simulink model "phan1_bai2a_kieu1_2016a"  (R2016a)
settings: Solver=VariableStepAuto  SolverMode=SingleTasking  StartTime=0.0  StopTime=30  RelTol=1e-3
libraries: simulink x1
settings Model: Creator=inhuo  LastModifiedBy=inhuo
settings DataIOCC: ReturnWorkspaceOutputs=on
settings DebuggingCC: SFUnexpectedBacktrackingDiag=error  SFNoUnconditionalDefaultTransitionDiag=error
settings SFSimCC: SimUseLocalCustomCode=on
settings RTWCC: RTWUseLocalCustomCode=on
settings GRTTargetCC: TargetLangStandard=C99 (ISO)  GeneratePreprocessorConditionals=Use local settings
settings ConfigComp: CovMetricSettings=dwe  CovHtmlReporting=off  CovSaveCumulativeToWorkspaceVar=off  CovSaveSingleToWorkspaceVar=off  CovExternalEMLEnable=on

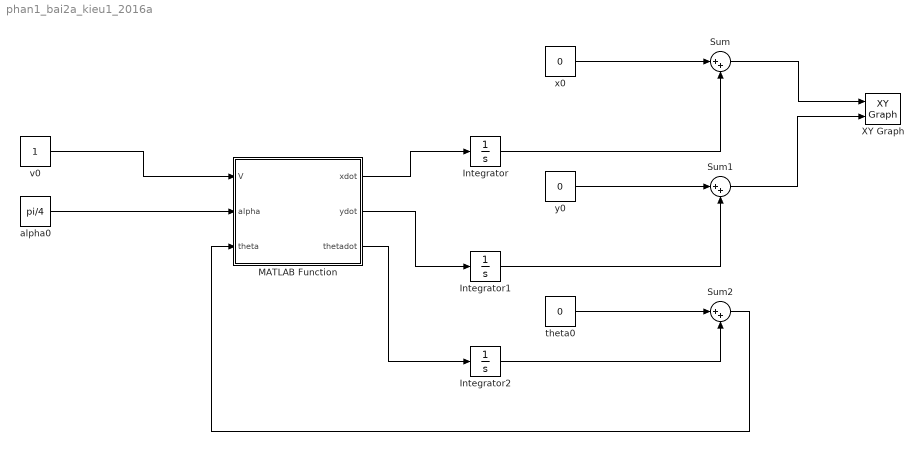
== system phan1_bai2a_kieu1_2016a ==
  Integrator : Integrator
  Integrator1 : Integrator
  Integrator2 : Integrator
  MATLAB Function : MATLAB Function  TreatAsAtomicUnit=on
  Sum : Sum  Inputs=|++
  Sum1 : Sum  Inputs=|++
  Sum2 : Sum  Inputs=|++
  XY Graph : simulink/Sinks/XY Graph  xmin=-5  xmax=10  ymin=-5  ymax=10  st=-1
  alpha0 : Constant  Value=pi/4
  theta0 : Constant  Value=0
  v0 : Constant
  x0 : Constant  Value=0
  y0 : Constant  Value=0
  wires:
  Sum2/1 -> MATLAB Function/3(theta)
  v0/1 -> MATLAB Function/1(V)
  MATLAB Function/2(ydot) -> Integrator1/1
  Sum/1 -> XY Graph/1
  Integrator1/1 -> Sum1/2
  MATLAB Function/3(thetadot) -> Integrator2/1
  x0/1 -> Sum/1
  Sum1/1 -> XY Graph/2
  theta0/1 -> Sum2/1
  Integrator2/1 -> Sum2/2
  y0/1 -> Sum1/1
  alpha0/1 -> MATLAB Function/2(alpha)
  MATLAB Function/1(xdot) -> Integrator/1
  Integrator/1 -> Sum/2

== matlab function phan1_bai2a_kieu1_2016a/MATLAB Function ==
  data: V input; xdot output; alpha input; theta input; ydot output; thetadot output
function [xdot , ydot , thetadot]= fcn(V,alpha,theta)

    d = sqrt (2.5 + 0.1*9);

    if abs(alpha)>pi/4
        alpha = pi/4*sign(alpha);
    end

    if V > (1.5 + 0.03 * 9) %lon hon van toc cuc dai
        V = (1.5 + 0.03 * 9)
    end
    % 
%     xdot = V*cos(theta);
%     ydot = V*sin(theta);
%     thetadot =V*tan(alpha)/d;
     %case 1 : kieu 1
     xdot = V*cos(alpha)*cos(theta);
     ydot = V*cos(alpha)*sin(theta);
     thetadot =V*sin(alpha)/d;
     
end


% case 1 
%      xdot = V*cos(alpha)*cos(theta);
%      ydot = V*cos(alpha)*sin(theta);
%      thetadot =V*sin(alpha)/d;

% case 2
% xdot = V*cos(theta);
% ydot = V*sin(theta);
% thetadot =V*tan(alpha)/d;
